simulink model "nelinearni_model_sim"  (R2020a)
settings: Solver=FixedStepAuto  StartTime=0.0  StopTime=sim_duration  FixedStep=1e-3  RelTol=1e-3
undefined symbols (not defined in the file): C, E, L, R, ue, x2e
settings Model: Creator=M & M  LastModifiedBy=M & M

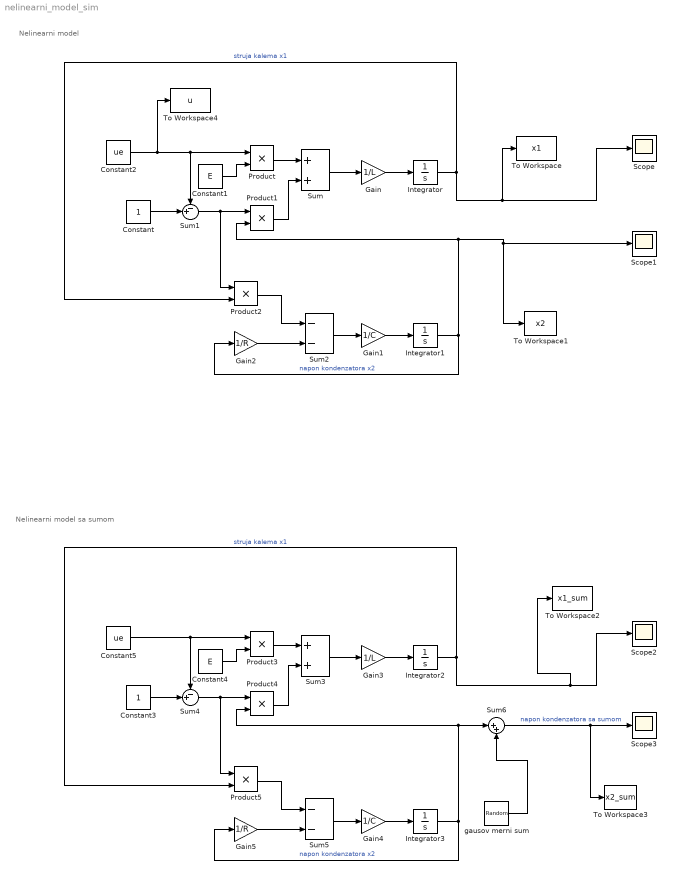
== system nelinearni_model_sim ==
  note: Nelinearni model sa sumom
  note: Nelinearni model
  Constant : Constant
  Constant1 : Constant  Value=E
  Constant2 : Constant  Value=ue
  Constant3 : Constant
  Constant4 : Constant  Value=E
  Constant5 : Constant  Value=ue
  Gain : Gain  Gain=1/L
  Gain1 : Gain  Gain=1/C
  Gain2 : Gain  Gain=1/R
  Gain3 : Gain  Gain=1/L
  Gain4 : Gain  Gain=1/C
  Gain5 : Gain  Gain=1/R
  Integrator{,1..3} (4 alike) : Integrator
  Product{,1..5} (6 alike) : Product
  Scope{,1..3} (4 alike) : Scope
  Sum : Sum
  Sum1 : Sum  Inputs=-+|
  Sum2 : Sum  Inputs=--
  Sum3 : Sum
  Sum4 : Sum  Inputs=-+|
  Sum5 : Sum  Inputs=--
  Sum6 : Sum  Inputs=|++
  To Workspace : ToWorkspace  VariableName=x1  SaveFormat=Timeseries  SampleTime=-1
  To Workspace1 : ToWorkspace  VariableName=x2  SaveFormat=Timeseries  SampleTime=-1
  To Workspace2 : ToWorkspace  VariableName=x1_sum  SaveFormat=Timeseries  SampleTime=-1
  To Workspace3 : ToWorkspace  VariableName=x2_sum  SaveFormat=Timeseries  SampleTime=-1
  To Workspace4 : ToWorkspace  VariableName=u  SampleTime=-1
  gausov merni sum : RandomNumber  Variance=(0.05*x2e)^2  SampleTime=0.1
  wires:
  Product2/1 -> Sum2/1
  Sum1/1 -> Product2/1, Product1/1
  Constant2/1 -> To Workspace4/1, Sum1/1, Product/1
  Product1/1 -> Sum/2
  Gain/1 -> Integrator/1
  Constant1/1 -> Product/2
  Sum/1 -> Gain/1
  Gain1/1 -> Integrator1/1
  Gain2/1 -> Sum2/2
  Product/1 -> Sum/1
  Sum2/1 -> Gain1/1
  Integrator/1 -> To Workspace/1, Scope/1, Product2/2  "struja kalema x1"
  Integrator1/1 -> Gain2/1, Product1/2, To Workspace1/1, Scope1/1  "napon kondenzatora x2"
  Constant/1 -> Sum1/2
  Constant3/1 -> Sum4/2
  Integrator2/1 -> To Workspace2/1, Scope2/1, Product5/2  "struja kalema x1"
  Integrator3/1 -> Gain5/1, Product4/2, Sum6/1  "napon kondenzatora x2"
  Product4/1 -> Sum3/2
  Gain5/1 -> Sum5/2
  Sum5/1 -> Gain4/1
  Gain3/1 -> Integrator2/1
  Sum4/1 -> Product5/1, Product4/1
  Product3/1 -> Sum3/1
  Constant4/1 -> Product3/2
  Product5/1 -> Sum5/1
  Gain4/1 -> Integrator3/1
  Constant5/1 -> Sum4/1, Product3/1
  Sum3/1 -> Gain3/1
  Sum6/1 -> To Workspace3/1, Scope3/1  "napon kondenzatora sa sumom"
  gausov merni sum/1 -> Sum6/2
